simulink model "staubli_20210324_v18a"  (R2018a)
settings: Solver=VariableStepAuto  StartTime=0.0  StopTime=10  RelTol=1e-3
libraries: dsppolyfun x6, simulink x6
settings Model: Creator=kdc95  LastModifiedBy=UNIST
settings SolverCC: ZeroCrossAlgorithm=Adaptive
settings DataIOCC: ReturnWorkspaceOutputs=on
settings DebuggingCC: IgnoredZcDiagnostic=none
settings SFSimCC: SimUseLocalCustomCode=on
settings RTWCC: RTWUseLocalCustomCode=on

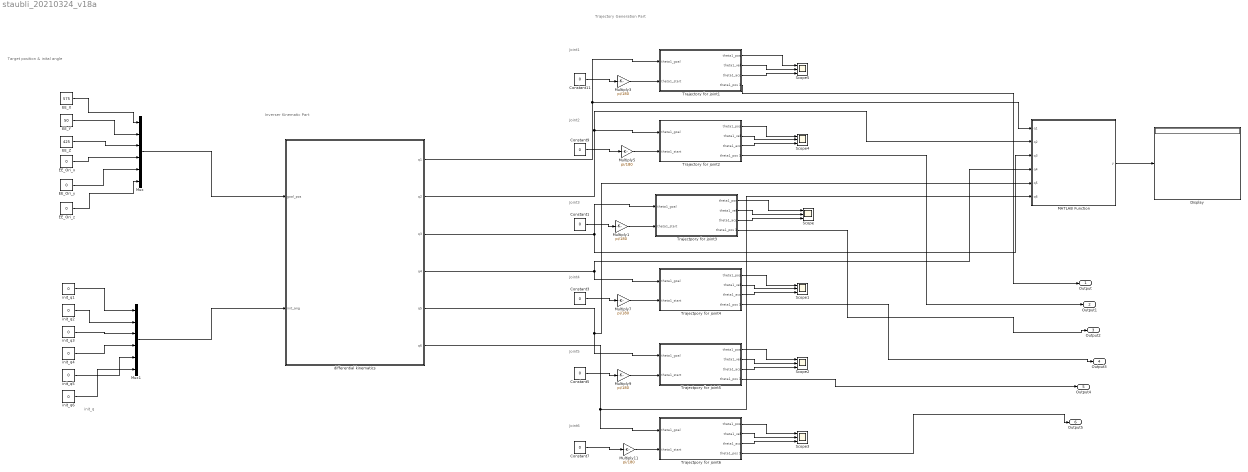
== system staubli_20210324_v18a ==
  note: Trajectory Generation Part
  note: init_q
  note: Joint2
  note: Joint3
  note: Joint4
  note: Joint5
  note: Joint1
  note: Joint6
  note: Target position & inital angle
  note: Inverser Kinematic Part
  Constant{1,3,5,7,9,11} (6 alike) : Constant  Value=0
  Display : Display
  EE_Ori_x : Constant  Value=0
  EE_Ori_y : Constant  Value=0
  EE_Ori_z : Constant  Value=0
  EE_X : Constant  Value=575
  EE_Y : Constant  Value=50
  EE_Z : Constant  Value=425
  MATLAB Function : MATLAB Function  TreatAsAtomicUnit=on
  Multiply{1,3,5,7,9,11} (6 alike) : Gain  Gain=pi/180
  Mux : Mux  Inputs=6
  Mux1 : Mux  Inputs=6
  Scope{,1..5} (6 alike) : Scope  NumInputPorts=3
  Trajectory for joint1 : Subsystem
  Trajectory for joint2 : Subsystem
  Trajectpory for joint3 : Subsystem
  Trajectpory for joint4 : Subsystem
  Trajectpory for joint5 : Subsystem
  Trajectpory for joint6 : Subsystem
  differential kinematics : Subsystem
  init_q{1..6} (6 alike) : Constant  Value=0
  Output : Outport
  Output1 : Outport  Port=2
  Output2 : Outport  Port=3
  Output3 : Outport  Port=4
  Output4 : Outport  Port=5
  Output5 : Outport  Port=6
  wires:
  Trajectpory for joint3/1("theta1_pos ") -> Scope/1
  Trajectory for joint1/3("theta1_acc ") -> Scope5/3
  Trajectpory for joint3/3("theta1_acc ") -> Scope/3
  Constant5/1 -> Multiply9/1
  Trajectpory for joint4/1("theta1_pos ") -> Scope1/1
  Constant11/1 -> Multiply3/1
  Trajectpory for joint5/2("theta1_vel ") -> Scope2/2
  Trajectpory for joint3/2("theta1_vel ") -> Scope/2
  Constant3/1 -> Multiply7/1
  Trajectory for joint1/2("theta1_vel ") -> Scope5/2
  Trajectpory for joint5/1("theta1_pos ") -> Scope2/1
  Trajectpory for joint6/1("theta1_pos ") -> Scope3/1
  Trajectpory for joint5/3("theta1_acc ") -> Scope2/3
  Constant7/1 -> Multiply11/1
  Trajectory for joint2/2("theta1_vel ") -> Scope4/2
  Trajectpory for joint6/3("theta1_acc ") -> Scope3/3
  Trajectory for joint2/1("theta1_pos ") -> Scope4/1
  Trajectory for joint2/3("theta1_acc ") -> Scope4/3
  Trajectpory for joint6/2("theta1_vel ") -> Scope3/2
  Constant1/1 -> Multiply1/1
  Constant9/1 -> Multiply5/1
  Trajectpory for joint4/2("theta1_vel ") -> Scope1/2
  Trajectpory for joint4/3("theta1_acc ") -> Scope1/3
  Trajectory for joint1/1("theta1_pos ") -> Scope5/1
  Trajectory for joint1/4(theta1_pos 1) -> Output/1
  Trajectory for joint2/4(theta1_pos 1) -> Output1/1
  Trajectpory for joint3/4(theta1_pos 1) -> Output2/1
  Trajectpory for joint4/4(theta1_pos 1) -> Output3/1
  Trajectpory for joint5/4(theta1_pos 1) -> Output4/1
  Trajectpory for joint6/4(theta1_pos 1) -> Output5/1
  differential kinematics/3(q3) -> Trajectpory for joint3/1("theta1_goal "), MATLAB Function/3(q3)
  Multiply1/1 -> Trajectpory for joint3/2("theta1_start ")
  differential kinematics/1(q1) -> Trajectory for joint1/1("theta1_goal "), MATLAB Function/1(q1)
  Multiply3/1 -> Trajectory for joint1/2("theta1_start ")
  differential kinematics/2(q2) -> Trajectory for joint2/1("theta1_goal "), MATLAB Function/2(q2)
  Multiply5/1 -> Trajectory for joint2/2("theta1_start ")
  differential kinematics/4(q4) -> MATLAB Function/4(q4), Trajectpory for joint4/1("theta1_goal ")
  Multiply7/1 -> Trajectpory for joint4/2("theta1_start ")
  differential kinematics/5(q5) -> Trajectpory for joint5/1("theta1_goal "), MATLAB Function/5(q5)
  Multiply9/1 -> Trajectpory for joint5/2("theta1_start ")
  differential kinematics/6(q6) -> Trajectpory for joint6/1("theta1_goal "), MATLAB Function/6(q6)
  Multiply11/1 -> Trajectpory for joint6/2("theta1_start ")
  MATLAB Function/1(y) -> Display/1
  EE_X/1 -> Mux/1
  EE_Y/1 -> Mux/2
  EE_Z/1 -> Mux/3
  EE_Ori_x/1 -> Mux/4
  EE_Ori_y/1 -> Mux/5
  EE_Ori_z/1 -> Mux/6
  init_q1/1 -> Mux1/1
  init_q2/1 -> Mux1/2
  init_q3/1 -> Mux1/3
  init_q4/1 -> Mux1/4
  init_q5/1 -> Mux1/5
  init_q6/1 -> Mux1/6
  Mux/1 -> differential kinematics/1(goal_pos)
  Mux1/1 -> differential kinematics/2(init_ang)

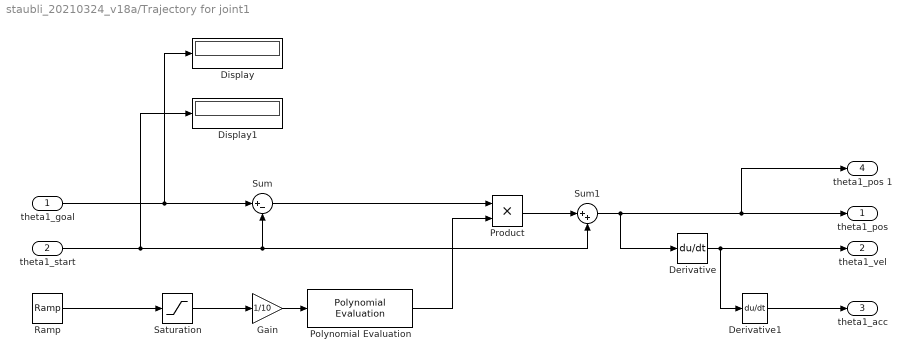
== system staubli_20210324_v18a/Trajectory for joint1 ==
  "theta1_goal " : Inport
  "theta1_start " : Inport  Port=2
  Derivative : Derivative
  Derivative1 : Derivative
  Display : Display
  Display1 : Display
  Gain : Gain  Gain=1/10
  Polynomial Evaluation : dsppolyfun/Polynomial Evaluation  useConstCoeffs=on  constCoeffs=[6 -15 10 0 0 0]
      settings: SourceProductBaseCode=DS
  Product : Product
  Ramp : simulink/Sources/Ramp  slope=1  start=0  InitialOutput=0
  Saturation : Saturate  UpperLimit=10  LowerLimit=-10
  Sum : Sum  Inputs=|+-
  Sum1 : Sum  Inputs=|++
  "theta1_pos " : Outport  VectorParamsAs1DForOutWhenUnconnected=off
  "theta1_vel " : Outport  Port=2  VectorParamsAs1DForOutWhenUnconnected=off
  "theta1_acc " : Outport  Port=3  VectorParamsAs1DForOutWhenUnconnected=off
  theta1_pos 1 : Outport  Port=4  VectorParamsAs1DForOutWhenUnconnected=off
  wires:
  "theta1_start "/1 -> Sum1/2, Sum/2, Display1/1
  Sum/1 -> Product/1
  "theta1_goal "/1 -> Display/1, Sum/1
  Sum1/1 -> Derivative/1, theta1_pos 1/1, "theta1_pos "/1
  Derivative/1 -> "theta1_vel "/1, Derivative1/1
  Gain/1 -> Polynomial Evaluation/1
  Product/1 -> Sum1/1
  Polynomial Evaluation/1 -> Product/2
  Derivative1/1 -> "theta1_acc "/1
  Saturation/1 -> Gain/1
  Ramp/1 -> Saturation/1

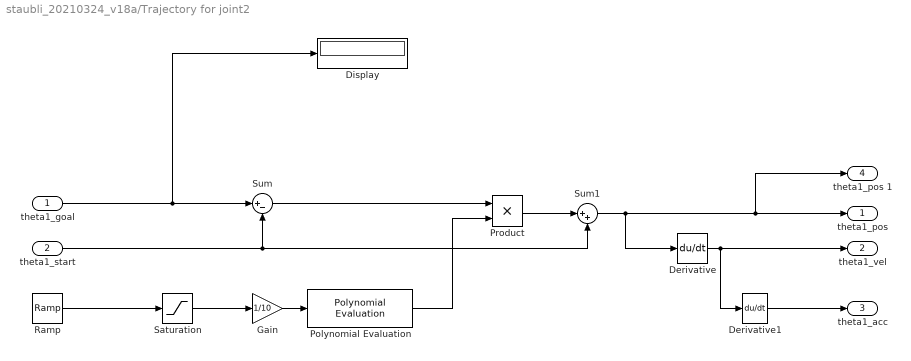
== system staubli_20210324_v18a/Trajectory for joint2 ==
  "theta1_goal " : Inport
  "theta1_start " : Inport  Port=2
  Derivative : Derivative
  Derivative1 : Derivative
  Display : Display
  Gain : Gain  Gain=1/10
  Polynomial Evaluation : dsppolyfun/Polynomial Evaluation  useConstCoeffs=on  constCoeffs=[6 -15 10 0 0 0]
      settings: SourceProductBaseCode=DS
  Product : Product
  Ramp : simulink/Sources/Ramp  slope=1  start=0  InitialOutput=0
  Saturation : Saturate  UpperLimit=10  LowerLimit=-10
  Sum : Sum  Inputs=|+-
  Sum1 : Sum  Inputs=|++
  "theta1_pos " : Outport  VectorParamsAs1DForOutWhenUnconnected=off
  "theta1_vel " : Outport  Port=2  VectorParamsAs1DForOutWhenUnconnected=off
  "theta1_acc " : Outport  Port=3  VectorParamsAs1DForOutWhenUnconnected=off
  theta1_pos 1 : Outport  Port=4  VectorParamsAs1DForOutWhenUnconnected=off
  wires:
  "theta1_start "/1 -> Sum1/2, Sum/2
  Sum/1 -> Product/1
  "theta1_goal "/1 -> Display/1, Sum/1
  Sum1/1 -> Derivative/1, theta1_pos 1/1, "theta1_pos "/1
  Derivative/1 -> "theta1_vel "/1, Derivative1/1
  Gain/1 -> Polynomial Evaluation/1
  Product/1 -> Sum1/1
  Polynomial Evaluation/1 -> Product/2
  Derivative1/1 -> "theta1_acc "/1
  Saturation/1 -> Gain/1
  Ramp/1 -> Saturation/1

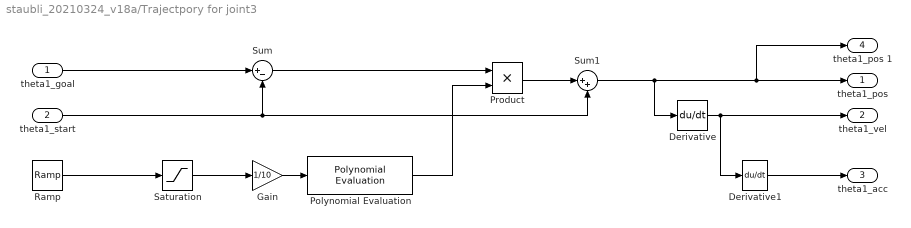
== system staubli_20210324_v18a/Trajectpory for joint3 ==
  "theta1_goal " : Inport
  "theta1_start " : Inport  Port=2
  Derivative : Derivative
  Derivative1 : Derivative
  Gain : Gain  Gain=1/10
  Polynomial Evaluation : dsppolyfun/Polynomial Evaluation  useConstCoeffs=on  constCoeffs=[6 -15 10 0 0 0]
      settings: SourceProductBaseCode=DS
  Product : Product
  Ramp : simulink/Sources/Ramp  slope=1  start=0  InitialOutput=0
  Saturation : Saturate  UpperLimit=10  LowerLimit=-10
  Sum : Sum  Inputs=|+-
  Sum1 : Sum  Inputs=|++
  "theta1_pos " : Outport  VectorParamsAs1DForOutWhenUnconnected=off
  "theta1_vel " : Outport  Port=2  VectorParamsAs1DForOutWhenUnconnected=off
  "theta1_acc " : Outport  Port=3  VectorParamsAs1DForOutWhenUnconnected=off
  theta1_pos 1 : Outport  Port=4  VectorParamsAs1DForOutWhenUnconnected=off
  wires:
  Sum/1 -> Product/1
  Derivative/1 -> "theta1_vel "/1, Derivative1/1
  Gain/1 -> Polynomial Evaluation/1
  Product/1 -> Sum1/1
  Polynomial Evaluation/1 -> Product/2
  Derivative1/1 -> "theta1_acc "/1
  Saturation/1 -> Gain/1
  Ramp/1 -> Saturation/1
  "theta1_goal "/1 -> Sum/1
  "theta1_start "/1 -> Sum1/2, Sum/2
  Sum1/1 -> Derivative/1, theta1_pos 1/1, "theta1_pos "/1

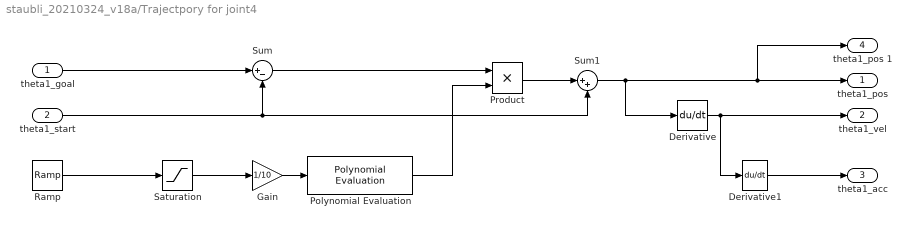
== system staubli_20210324_v18a/Trajectpory for joint4 ==
  "theta1_goal " : Inport
  "theta1_start " : Inport  Port=2
  Derivative : Derivative
  Derivative1 : Derivative
  Gain : Gain  Gain=1/10
  Polynomial Evaluation : dsppolyfun/Polynomial Evaluation  useConstCoeffs=on  constCoeffs=[6 -15 10 0 0 0]
      settings: SourceProductBaseCode=DS
  Product : Product
  Ramp : simulink/Sources/Ramp  slope=1  start=0  InitialOutput=0
  Saturation : Saturate  UpperLimit=10  LowerLimit=-10
  Sum : Sum  Inputs=|+-
  Sum1 : Sum  Inputs=|++
  "theta1_pos " : Outport  VectorParamsAs1DForOutWhenUnconnected=off
  "theta1_vel " : Outport  Port=2  VectorParamsAs1DForOutWhenUnconnected=off
  "theta1_acc " : Outport  Port=3  VectorParamsAs1DForOutWhenUnconnected=off
  theta1_pos 1 : Outport  Port=4  VectorParamsAs1DForOutWhenUnconnected=off
  wires:
  "theta1_start "/1 -> Sum1/2, Sum/2
  Sum/1 -> Product/1
  "theta1_goal "/1 -> Sum/1
  Sum1/1 -> Derivative/1, theta1_pos 1/1, "theta1_pos "/1
  Derivative/1 -> "theta1_vel "/1, Derivative1/1
  Gain/1 -> Polynomial Evaluation/1
  Product/1 -> Sum1/1
  Polynomial Evaluation/1 -> Product/2
  Derivative1/1 -> "theta1_acc "/1
  Saturation/1 -> Gain/1
  Ramp/1 -> Saturation/1

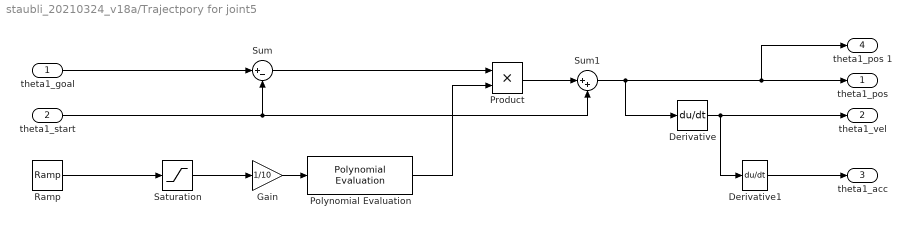
== system staubli_20210324_v18a/Trajectpory for joint5 ==
  "theta1_goal " : Inport
  "theta1_start " : Inport  Port=2
  Derivative : Derivative
  Derivative1 : Derivative
  Gain : Gain  Gain=1/10
  Polynomial Evaluation : dsppolyfun/Polynomial Evaluation  useConstCoeffs=on  constCoeffs=[6 -15 10 0 0 0]
      settings: SourceProductBaseCode=DS
  Product : Product
  Ramp : simulink/Sources/Ramp  slope=1  start=0  InitialOutput=0
  Saturation : Saturate  UpperLimit=10  LowerLimit=-10
  Sum : Sum  Inputs=|+-
  Sum1 : Sum  Inputs=|++
  "theta1_pos " : Outport  VectorParamsAs1DForOutWhenUnconnected=off
  "theta1_vel " : Outport  Port=2  VectorParamsAs1DForOutWhenUnconnected=off
  "theta1_acc " : Outport  Port=3  VectorParamsAs1DForOutWhenUnconnected=off
  theta1_pos 1 : Outport  Port=4  VectorParamsAs1DForOutWhenUnconnected=off
  wires:
  "theta1_start "/1 -> Sum1/2, Sum/2
  Sum/1 -> Product/1
  "theta1_goal "/1 -> Sum/1
  Sum1/1 -> Derivative/1, theta1_pos 1/1, "theta1_pos "/1
  Derivative/1 -> "theta1_vel "/1, Derivative1/1
  Gain/1 -> Polynomial Evaluation/1
  Product/1 -> Sum1/1
  Polynomial Evaluation/1 -> Product/2
  Derivative1/1 -> "theta1_acc "/1
  Saturation/1 -> Gain/1
  Ramp/1 -> Saturation/1

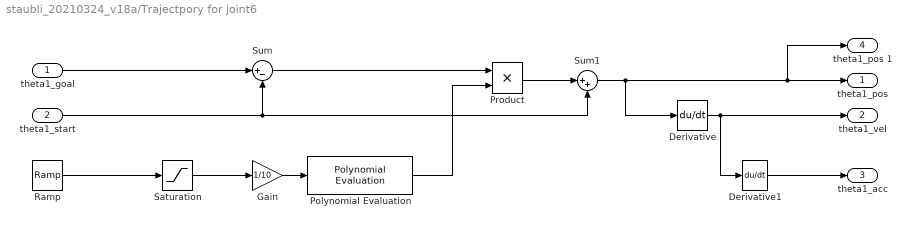
== system staubli_20210324_v18a/Trajectpory for joint6 ==
  "theta1_goal " : Inport
  "theta1_start " : Inport  Port=2
  Derivative : Derivative
  Derivative1 : Derivative
  Gain : Gain  Gain=1/10
  Polynomial Evaluation : dsppolyfun/Polynomial Evaluation  useConstCoeffs=on  constCoeffs=[6 -15 10 0 0 0]
      settings: SourceProductBaseCode=DS
  Product : Product
  Ramp : simulink/Sources/Ramp  slope=1  start=0  InitialOutput=0
  Saturation : Saturate  UpperLimit=20  LowerLimit=-20
  Sum : Sum  Inputs=|+-
  Sum1 : Sum  Inputs=|++
  "theta1_pos " : Outport  VectorParamsAs1DForOutWhenUnconnected=off
  "theta1_vel " : Outport  Port=2  VectorParamsAs1DForOutWhenUnconnected=off
  "theta1_acc " : Outport  Port=3  VectorParamsAs1DForOutWhenUnconnected=off
  theta1_pos 1 : Outport  Port=4  VectorParamsAs1DForOutWhenUnconnected=off
  wires:
  "theta1_start "/1 -> Sum1/2, Sum/2
  Sum/1 -> Product/1
  "theta1_goal "/1 -> Sum/1
  Sum1/1 -> Derivative/1, theta1_pos 1/1, "theta1_pos "/1
  Derivative/1 -> "theta1_vel "/1, Derivative1/1
  Gain/1 -> Polynomial Evaluation/1
  Product/1 -> Sum1/1
  Polynomial Evaluation/1 -> Product/2
  Derivative1/1 -> "theta1_acc "/1
  Saturation/1 -> Gain/1
  Ramp/1 -> Saturation/1

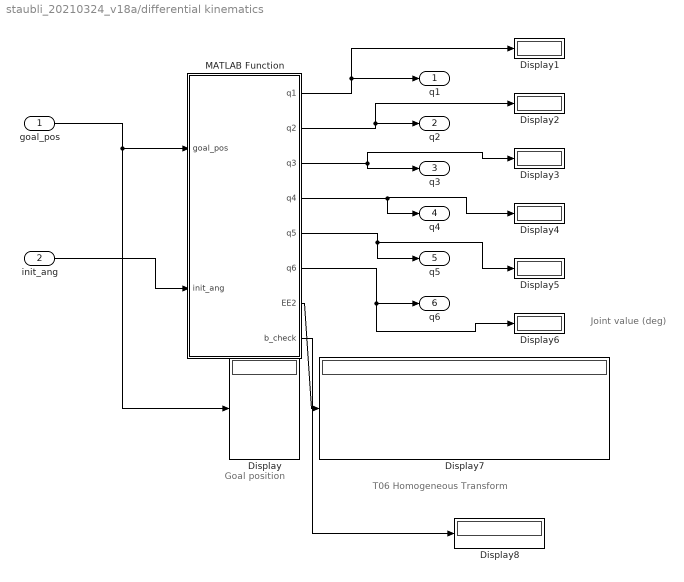
== system staubli_20210324_v18a/differential kinematics ==
  note: Joint value (deg)
  note: T06 Homogeneous Transform
  note: Goal position
  goal_pos : Inport
  init_ang : Inport  Port=2
  Display{,1..8} (9 alike) : Display
  MATLAB Function : MATLAB Function  TreatAsAtomicUnit=on
  q1 : Outport
  q2 : Outport  Port=2
  q3 : Outport  Port=3
  q4 : Outport  Port=4
  q5 : Outport  Port=5
  q6 : Outport  Port=6
  wires:
  goal_pos/1 -> Display/1, MATLAB Function/1(goal_pos)
  init_ang/1 -> MATLAB Function/2(init_ang)
  MATLAB Function/2(q2) -> Display2/1, q2/1
  MATLAB Function/3(q3) -> q3/1, Display3/1
  MATLAB Function/4(q4) -> Display4/1, q4/1
  MATLAB Function/5(q5) -> q5/1, Display5/1
  MATLAB Function/6(q6) -> Display6/1, q6/1
  MATLAB Function/1(q1) -> Display1/1, q1/1
  MATLAB Function/7(EE2) -> Display7/1
  MATLAB Function/8(b_check) -> Display8/1

== matlab function staubli_20210324_v18a/differential kinematics/MATLAB Function ==
  data: goal_pos input; q1 output; init_ang input; q2 output; q3 output; q4 output; q5 output; q6 output; EE2 output; b_check output
function [q1,q2, q3, q4, q5, q6, EE2,b_check]= jacobian(goal_pos, init_ang)
theta1=init_ang(1);  d1=478;   a1=0;  alpha1=-90; %parameter link1
theta2=init_ang(2);  d2=0;   a2=50;  alpha2=0; %parameter link2
theta3=init_ang(3);  d3=50;  a3=425;  alpha3=0; %parameter link3
theta4=init_ang(4);  d4=0;   a4=0;  alpha4=90; %parameter link4
theta5=init_ang(5);  d5=425; a5=0;  alpha5=0; %parameter link5
theta6=init_ang(6);  d6=100; a6=0;  alpha6=0; %parameter link6
offset2 = -90;
offset3 = 90;
% DH paramter 
End_EE = [0 0 0 0;
         0 0 0 0;
         0 0 0 0;
         0 0 0 1];
     
Xc=goal_pos(1);Yc=goal_pos(2);Zc=goal_pos(3);
r=goal_pos(4);p=goal_pos(5);yaw=goal_pos(6);
% init pos and orientation(Euler)

iteration = 0;
b = 0 ;
deltatheta1=0;deltatheta2=0; deltatheta3=0; %theta1,2,3 velocity
deltatheta4=0;deltatheta5=0; deltatheta6=0; %theta1,2,3 velocity
while b == 0
    if theta1 >180
        theta1 = -180 + theta1;
    elseif theta1 <-180
        theta1 = -theta1;
    end
    if theta2 >147.5
        theta2 = -147.5 + theta2;
    elseif theta2 <-130
        theta2 = -theta2;
    end
    if theta3 >145
        theta3 = -145 + theta3;
    elseif theta3 <-145
        theta3 = -theta3;
    end
    if theta4 >270
        theta4 = -270 + theta4;
    elseif theta4 <-270
        theta4 = -theta4;
    end
    if theta5 >140
        theta5 = -140 + theta5;
    elseif theta5 <-115
        theta5 = -theta5;
    end
    if theta6 >270
        theta6 = -270 + theta6;
    elseif theta6 <-270
        theta6 = -theta6;
    end
    result = [theta1 theta2 theta3 theta4 theta5 theta6]
    disp(result)
    theta1=theta1+deltatheta1/2;
    theta2=theta2+deltatheta2/2;
    theta3=theta3+deltatheta3/2;
    theta4=theta4+deltatheta4/2;
    theta5=theta5+deltatheta5/2;
    theta6=theta6+deltatheta6/2;
    if(iteration > 1000)
        % avoid too many calculation
        b=1;
        iteration = 0;
    end
    T01=[cosd(theta1) -cosd(alpha1)*sind(theta1) sind(alpha1)*sind(theta1) a1*cosd(theta1);
        sind(theta1) cosd(alpha1)*cosd(theta1)  -sind(alpha1)*cosd(theta1) a1*sind(theta1);
        0,sind(alpha1),cosd(alpha1),d1;
        0,0,0,1];
    T12=[cosd(theta2+offset2) -cosd(alpha2)*sind(theta2+offset2) sind(alpha2)*sind(theta2+offset2) a2*cosd(theta2+offset2);
        sind(theta2+offset2) cosd(alpha2)*cosd(theta2+offset2)  -sind(alpha2)*cosd(theta2+offset2) a2*sind(theta2+offset2);
        0,sind(alpha2),cosd(alpha2),d2;
        0,0,0,1];
    T23=[cosd(theta3+offset3) -cosd(alpha3)*sind(theta3+offset3) sind(alpha3)*sind(theta3+offset3) a3*cosd(theta3+offset3);
        sind(theta3+offset3) cosd(alpha3)*cosd(theta3+offset3)  -sind(alpha3)*cosd(theta3+offset3) a3*sind(theta3+offset3);
        0,sind(alpha3),cosd(alpha3),d3;
        0,0,0,1];
    T34=[cosd(theta4) -cosd(alpha4)*sind(theta4) sind(alpha4)*sind(theta4) a4*cosd(theta4);
         sind(theta4) cosd(alpha4)*cosd(theta4)  -sind(alpha4)*cosd(theta4) a4*sind(theta4);
         0,sind(alpha4),cosd(alpha4),d4;
         0,0,0,1];
    T45=[cosd(theta5) -cosd(alpha5)*sind(theta5) sind(alpha5)*sind(theta5) a5*cosd(theta5);
         sind(theta5) cosd(alpha5)*cosd(theta5)  -sind(alpha5)*cosd(theta5) a5*sind(theta5);
         0,sind(alpha5),cosd(alpha5),d5;
         0,0,0,1];
    T56=[cosd(theta6) -cosd(alpha6)*sind(theta6) sind(alpha6)*sind(theta6) a6*cosd(theta6);
         sind(theta6) cosd(alpha6)*cosd(theta6)  -sind(alpha6)*cosd(theta6) a6*sind(theta6);
         0,sind(alpha6),cosd(alpha6),d6;
         0,0,0,1];
    T01;
    T02 = T01*T12;
    T03=T01*T12*T23;
    T04=T01*T12*T23*T34;
    T05=T01*T12*T23*T34*T45;
    T06=T01*T12*T23*T34*T45*T56

    P0=[0 0 0];
    P1=transpose(T01(1:3,4));
    P2=transpose(T02(1:3,4));
    P3=transpose(T03(1:3,4));
    P4=transpose(T04(1:3,4));
    P5=transpose(T05(1:3,4));
    P6=transpose(T06(1:3,4));
    %%%%%%%%%%%%%%%%%%%%%%%
    Z0  = [0;0;1];Ori =[0;0;0]; O6=T06(1:3,4);
    Jv1 = cross(Z0,(O6-Ori));
    
    Z1  = T01(1:3,3);Ori_1=T01(1:3,4);
    Jv2 = cross(Z1,(O6-Ori_1));
    
    Z2  = T12(1:3,3);Ori_2=T12(1:3,4);
    Jv3 = cross(Z2,(O6-Ori_2));

    Z3  = T23(1:3,3);Ori_3=T23(1:3,4);
    Jv4 = cross(Z3,(O6-Ori_3));
    
    Z4  = T34(1:3,3);Ori_4=T34(1:3,4);
    Jv5 = cross(Z4,(O6-Ori_4));
    
    Z5  = T45(1:3,3);Ori_5=T45(1:3,4);
    Jv6 = cross(Z5,(O6-Ori_5));
    
    Jv=[Jv1 Jv2 Jv3 Jv4 Jv5 Jv6];

    Xinit=P6(1,1); 
    Yinit=P6(1,2);
    Zinit = P6(1,3);
    Xend=Xc;Yend=Yc; Zend = Zc;
    Xspeed=(Xend-Xinit);
    Yspeed=(Yend-Yinit);
    Zspeed=(Zend-Zinit);
    thetadot=pinv(Jv)*[Xspeed;Yspeed;Zspeed];
    error_x = Xspeed^2;
    error_z = Yspeed^2;
    error_y = Zspeed^2;
    dis_error=sqrt(error_x+error_y+error_z);
    
    if abs(error_x)<=0.2 && abs(error_y)<=0.2 && abs(error_z)<=0.2
        End_EE = T06;
        b=1;
    end
    theta1dot=thetadot(1,1);
    theta2dot=thetadot(2,1);
    theta3dot=thetadot(3,1);    
    theta4dot=thetadot(4,1);
    theta5dot=thetadot(5,1);
    theta6dot=thetadot(6,1);   
    
    deltatheta1=rad2deg(theta1dot);
    deltatheta2=rad2deg(theta2dot);
    deltatheta3=rad2deg(theta3dot);
    deltatheta4=rad2deg(theta4dot);
    deltatheta5=rad2deg(theta5dot);
    deltatheta6=rad2deg(theta6dot);
    iteration = iteration +1;
end
q1 = theta1;
q2 = theta2;
q3 = theta3;
q4 = theta4;
q5 = theta5;
q6 = theta6;
EE2 = End_EE;
b_check = b;

== matlab function staubli_20210324_v18a/MATLAB Function ==
  data: q1 input; y output; q2 input; q3 input; q4 input; q5 input; q6 input
function y = fcn(q1,q2,q3,q4,q5,q6)

y=[q1,q2,q3,q4,q5,q6];
% % y= [q1,q2,q3,q4,q5,q6]
% d1=0.1;
% d2=0.1;
% d3=0.1;
% d4=0.1;
% d5=0.1;
% d6=0.1;
% % 
% % 
% % q1=0;
% % q2=0;
% % q3=pi/2;
% % q4=0;
% % q5=0;
% % q6=0;
% 
% q0 = 0; %% base 부터 joint1 까지 거리 
% e0 = 0; %% endeffector wrist 부터 flange 까지 거리
% tcpx = 0; %% flange 부터 tcp 까지 거리
% tcpz = 0; %% flange 부터 tcp 까지 거리
% R = 0; %% TCP 각도 0
% 
% dq1=0;
% dq2=0;
% dq3=0;
% dq4=0;
% dq5=0;
% dq6=0;
% 
% 
% 
% % l1=0.0595-0.01;%doesnt matter
% l2=0.05;
% l3=0.0506;
% l4=0.0493;
% l5=0.0507;
% l6=0.05;
% 
% m1=1.4058;
% m2=1.2209;
% m3=0.9742;
% m4=0.7446;
% m5=0.7446;
% m6=0.3853;
% 
% zz1=0.000406218509370527;
% 
% xx2=0.000311258660573173;
% yy2=0.00113057980116099;
% zz2=0.00113500164711486;
% 
% xx3=0.000195610120509242;
% yy3=0.000890675212348444;
% zz3=0.000892205392556534;
% 
% xx4=0.000661301749537305;
% yy4=0.000114515268992527;
% zz4=0.000662306036923719;
% 
% xx5=0.000661293830235689;
% yy5=0.000114514748053103;
% zz5=0.000662295948156026;
% 
% xx6=0.000336151788940896; 
% yy6=0.000336151788940896;
% zz6=3.01034757383826E-05;
% 
% % syms q0 e0 tcpx tcpz R
% % syms q1 q2 q3 q4 q5 q6
% % syms d1 d2 d3 d4 d5 d6
% g = 9.8;
% 
% T1=[cos(q1)  0  sin(q1) 0;
%     sin(q1)  0 -cos(q1) 0;
%     0        1       0  d1;
%     0        0       0   1];
% 
% T2=[cos(q2) -sin(q2) 0 d2*cos(q2);
%     sin(q2)  cos(q2) 0 d2*sin(q2);
%     0              0 1          0;
%     0              0 0          1];
% 
% T3=[cos(q3) 0 sin(q3)  d3*cos(q3);
%     sin(q3) 0 -cos(q3) d3*sin(q3);
%     0       1  0          0;
%     0       0  0          1];
% 
% T4=[cos(q4) 0 -sin(q4)  0;
%     sin(q4) 0 cos(q4)   0;
%     0       1   0       d4;
%     0       0   0       1];
% 
% T5=[cos(q5) 0 -sin(q5)  d5*cos(q5);
%     sin(q5) 0 cos(q5)   d5*sin(q5);
%     0       1  0        0;
%     0       0   0       1];
% 
% T6=[cos(q6) -sin(q6) 0  0;
%     sin(q6)  cos(q6) 0  0;
%     0           0    1  d6;
%     0           0    0  1];
% 
% Tb = [1 0 0  0;
%     0  1 0  0;
%     0  0 1  q0;
%     0  0 0  1];
% 
% Tee = [1 0 0  0;
%     0  1 0  0;
%     0  0 1  e0;
%     0  0 0  1];
% 
% Ttcp = [cos(R) 0 sin(R)  tcpx;
%     0  1 0  0;
%     -sin(R)  0 cos(R)  tcpz;
%     0  0 0  1];
%    
% T01=T1;
% T02=T1*T2;
% T03=T1*T2*T3;
% T04=T1*T2*T3*T4;
% T05=T1*T2*T3*T4*T5;
% T06=T1*T2*T3*T4*T5*T6;
% Ttcp=Tb*T06*Tee*Ttcp;
% 
% R1=[cos(q1) -sin(q1) 0; %% the i th link rotation matrix
%     sin(q1)  cos(q1) 0;
%     0           0    1];
% 
% R2=[T02(1,1:3);
%     T02(2,1:3);
%     T02(3,1:3)];
% 
% R3=[T03(1,1:3);
%     T03(2,1:3);
%     T03(3,1:3)];
% 
% R4=[T04(1,1:3);
%     T04(2,1:3);
%     T04(3,1:3)];
% 
% R5=[T05(1,1:3);
%     T05(2,1:3);
%     T05(3,1:3)];
% 
% R6=[T06(1,1:3);
%     T06(2,1:3);
%     T06(3,1:3)];
% 
% jv1=jacobian([T01(1,4),T01(2,4),T01(3,4)],[q1,q2,q3,q4,q5,q6]);
% jv2=jacobian([T02(1,4),T02(2,4),T02(3,4)],[q1,q2,q3,q4,q5,q6]);
% jv3=jacobian([T03(1,4),T03(2,4),T03(3,4)],[q1,q2,q3,q4,q5,q6]);
% jv4=jacobian([T04(1,4),T04(2,4),T04(3,4)],[q1,q2,q3,q4,q5,q6]);
% jv5=jacobian([T05(1,4),T05(2,4),T05(3,4)],[q1,q2,q3,q4,q5,q6]);
% jv6=jacobian([T06(1,4),T06(2,4),T06(3,4)],[q1,q2,q3,q4,q5,q6]);
% % 
% % syms l1 l2 l3 l4 l5 l6
% 
% JV1=[0 0 0 0 0 0;  %% upper part of jacobian matrix
%      0 0 0 0 0 0;
%      0 0 0 0 0 0];
%   
% JV2=[-l2*cos(q2)*sin(q1), -l2*cos(q1)*sin(q2),0,0,0,0;
%       l2*cos(q1)*cos(q2), -l2*sin(q1)*sin(q2),0,0,0,0;
%                        0,          l2*cos(q2),0,0,0,0];
% 
% JV3=subs(jv3,d3,l3);
% JV4=subs(jv4,d4,l4);
% JV5=subs(jv5,d5,l5);
% JV6=subs(jv6,d6,l6);
% 
% jw=[0,T1(1,3),T02(1,3),T03(1,3),T04(1,3),T05(1,3);  %% lower part of jacobian
%     0,T1(2,3),T02(2,3),T03(2,3),T04(2,3),T05(2,3);
%     1,T1(3,3),T02(3,3),T03(3,3),T04(3,3),T05(3,3)];
% 
% JW1=jw;
% JW1(:,2:6)=0;
% 
% JW2=jw;
% JW2(:,3:6)=0;
% 
% JW3=jw;
% JW3(:,4:6)=0;
% 
% JW4=jw;
% JW4(:,5:6)=0;
% 
% JW5=jw;
% JW5(:,6)=0;
% 
% JW6=jw;
% 
% % syms m1 m2 m3 m4 m5 m6
% % syms xx1 yy1 zz1 xx2 yy2 zz2 xx3 yy3 zz3
% % syms xx4 yy4 zz4 xx5 yy5 zz5 xx6 yy6 zz6
% 
% IXX=[xx1 xx2 xx3 xx4 xx5 xx6];
% IYY=[yy1 yy2 yy3 yy4 yy5 yy6];
% IZZ=[zz1 zz2 zz3 zz4 zz5 zz6];
% 
% I1=[IXX(1) 0 0; 0 IYY(1) 0; 0 0 IZZ(1)]; %% inertia tensor
% I2=[IXX(2) 0 0; 0 IYY(2) 0; 0 0 IZZ(2)];
% I3=[IXX(3) 0 0; 0 IYY(3) 0; 0 0 IZZ(3)];
% I4=[IXX(4) 0 0; 0 IYY(4) 0; 0 0 IZZ(4)];
% I5=[IXX(5) 0 0; 0 IYY(5) 0; 0 0 IZZ(5)];
% I6=[IXX(6) 0 0; 0 IYY(6) 0; 0 0 IZZ(6)];
% 
% D1=m1*JV1.'*JV1+JW1.'*R1*I1*R1.'*JW1; %% joint-space inertia matrix
% D2=m2*JV2.'*JV2+JW2.'*R2*I2*R2.'*JW2;
% D3=m3*JV3.'*JV3+JW3.'*R3*I3*R3.'*JW3;
% D4=m4*JV4.'*JV4+JW4.'*R4*I4*R4.'*JW4;
% D5=m5*JV5.'*JV5+JW5.'*R5*I5*R5.'*JW5;
% D6=m6*JV6.'*JV6+JW6.'*R6*I6*R6.'*JW6;
% 
% 
% D=D1+D2+D3+D4+D5+D6;
% % 
% % syms dq1 dq2 dq3 dq4 dq5 dq6
% 
% Q=[q1 q2 q3 q4 q5 q6]
% DQ=[dq1 dq2 dq3 dq4 dq5 dq6]
% C=sym(zeros(6)); %% Christoffel matrix, which presents the centrifugal and Coriolis terms
% for k=1:6
%     for j=1:6
%         for i=1:6
%             C(k,j)=C(k,j)+(1/2*(diff(D(k,j),Q(i))+jacobian(D(k,i),Q(j))-jacobian(D(i,j),Q(k))))*DQ(i);
%         end
%         
%     end
% end
% 
% %  % seeking gravity matrix
% %  P1 =[x1;y1;z1]; % the coordinates of centroid 1 at {1}
% %  P01 = T01([1 2 3],[1 2 3])*P1; % centroid 1 is under {0}
% % 
% %  P2 = [x2; y2; z2]; % centroid 2 at {2} coordinates
% %  P02 = T02([1 2 3],[1 2 3])*P2; % centroid 2 coordinates in {0}
% % 
% %  P3 = [x3; y3; z3]; % centroid 3 at {3} coordinates
% %  P03 = T03([1 2 3], [1 2 3])*P3; % centroid 3 coordinates in {0}
% % 
% %  P4 = [x4; y4; z4]; %coordinates of  centroid 4 at {4}
% % P04 = T04([1 2 3],[1 2 3])*P4; % centroid 4 is under {0}
% % 
% %  P5 = [x5; y5; z5]; % centroid 5 at {5} coordinates
% %  P05 = T05([1 2 3],[1 2 3])*P5; % centroid 5 is under {0}
% % 
% %  P6 = [x1; y1; z1]; %the coordinates of % centroid 6 at {6}
% %  P06 = T06([1 2 3],[1 2 3])*P6; % centroid 6 is under {0}
% % 
% %  % potential expression
% % P = m1*g*P01(3,1)+m2*g*P02(3,1)+m3*g*P03(3,1)+m4*g*P04(3,1)+m5*g*P05(3,1)+m6*g*P06(3,1);
% % 
% %  % potential can be used to guide theta1
% % G01 = diff( P,q1);
% %  % potential can be used to guide theta2
% % G02 = diff( P,q2);
% %  % potential can be used to guide theta3
% % G03 = diff( P,q3);
% %  % potential can be used to guide theta4
% % G04 = diff( P,q4);
% %  % potential can be partial to theta5
% % G05 = diff( P,q5);
% %  % potential can be used to guide theta6
% % G06 = diff( P,q6);
% % 
% %  % gravity matrix
% % G = [G01; G02; G03; G04; G05; G06];
% 
% 
% M=subs(D)
% JV=subs(jv6)
% 
% K=eye(6)*100
% range=1000;
% for tmp=1:1:range 
%     
%     w=tmp*2*pi;
%     
%     G=M*(-w^2)+K;
%   
%     FRF=JV*inv(G)*JV.';
%     
%     hxx=abs(FRF(1,1));
%     hxy=abs(FRF(2,1));
%     hxz=abs(FRF(3,1));
%     
%     hyy=abs(FRF(2,2));
%     hyz=abs(FRF(3,2));
%     
%     hzz=abs(FRF(3,3));
%     
%     
% end
% 
% 
%     plot(1:range,hxx(1:range))
%     grid on
%     legend('model','FEM') 
%     set(gca, 'YScale', 'log')
%     textobj = findobj('type', 'axes');
%             set(textobj, 'fontname', 'Times New Roman');
%             set(textobj, 'fontunits', 'points');
%             set(textobj, 'fontsize', 16);
%             set(textobj,'fontweight','bold');
%             xlim([0 500]);
% 
%     title('h_{ffxx}')
%     xlabel('frequency (Hz)')
%     ylabel('magnitude (m/N)')
% 
%     figure
%     plot(1:range,hxy(1:range))
%     grid on
%     legend('model','FEM')
%     set(gca, 'YScale', 'log')
%     textobj = findobj('type', 'axes');
%             set(textobj, 'fontname', 'Times New Roman');
%             set(textobj, 'fontunits', 'points');
%             set(textobj, 'fontsize', 16);
%             set(textobj,'fontweight','bold');
%             xlim([0 1000]);
% 
%     title('h_{ffxy}')
%     xlabel('frequency (Hz)')
%     ylabel('magnitude (m/N)')
%     
%     figure
%     plot(1:range,hxz(1:range))
%     grid on
%     legend('model','FEM')
%     set(gca, 'YScale', 'log')
%     textobj = findobj('type', 'axes');
%             set(textobj, 'fontname', 'Times New Roman');
%             set(textobj, 'fontunits', 'points');
%             set(textobj, 'fontsize', 16);
%             set(textobj,'fontweight','bold');
%             xlim([0 1000]);
% 
%     title('h_{ffxz}')
%     xlabel('frequency (Hz)')
%     ylabel('magnitude (m/N)')
% 
%     figure
%     plot(1:range,hyy(1:range))
%     grid on
%     legend('model','FEM')
%     set(gca, 'YScale', 'log')
%     textobj = findobj('type', 'axes');
%             set(textobj, 'fontname', 'Times New Roman');
%             set(textobj, 'fontunits', 'points');
%             set(textobj, 'fontsize', 16);
%             set(textobj,'fontweight','bold');
%             xlim([0 1000]);
% 
%     title('h_{ffyy}')
%     xlabel('frequency (Hz)')
%     ylabel('magnitude (m/N)')
%     
%     figure
%     plot(1:range,hyz(1:range))
%     grid on
%     legend('model','FEM')
%     set(gca, 'YScale', 'log')
%     textobj = findobj('type', 'axes');
%             set(textobj, 'fontname', 'Times New Roman');
%             set(textobj, 'fontunits', 'points');
%             set(textobj, 'fontsize', 16);
%             set(textobj,'fontweight','bold');
%             xlim([0 1000]);
% 
%     title('h_{ffyz}')
%     xlabel('frequency (Hz)')
%     ylabel('magnitude (m/N)')
% 
%     figure
%     plot(1:range,hzz(1:range))
%     grid on
%     legend('model','FEM')
%     set(gca, 'YScale', 'log')
%     textobj = findobj('type', 'axes');
%             set(textobj, 'fontname', 'Times New Roman');
%             set(textobj, 'fontunits', 'points');
%             set(textobj, 'fontsize', 16);
%             set(textobj,'fontweight','bold');
%             xlim([0 1000]);
% 
%     title('h_{ffzz}')
%     xlabel('frequency (Hz)')
%     ylabel('magnitude (m/N)')
% 
% 
% y = q1;
